simulink model "WK_Maobi_writingDTP25"  (Simulink 7.7)
settings: Solver=ode4  StartTime=0.0  StopTime=inf  FixedStep=sample_time  RelTol=1e-3
InitFcn:
  | sample_time=0.005;%0.004;%0.0025;%0.02;
  | DeltaT = 0.02;
  | g = 9.81;
  | H0 = g%0.3165;
  | Kl = 1;
  | 
  | Omega_r = 1.6;%for Horizontal reference
  | Zeta_r = 0.7; %for Horizontal reference
  | Omega = 1.8;%for Horizontal Control
  | Zeta = 0.5;    %for Horizontal Control
  | 
  | Omega_h_r = 2.5; %for vertical reference
  | Zeta_h_r = 0.8;  %for vertical reference
  | Omega_h = 2.7;    %for vertical control
  | Zeta_h = 0.8;         %for vertical control
  | PI=pi;
  | 
  | Mass = 1.15;
  | Acc_Max = 4;
  | Acc_Max_h = 4;
  | 
  | Max_RP = 60;
  | 
  | % for NN
  | n = 5;
  | r = 3;
  | n2 = 5;
  | NN_ST = 0.02;
  | 
  | GAMA_V = 6;
  | gama_V_e = 0.01;
  | 
  | GAMA_W = GAMA_V;
  | gama_W_e =0.01;
  | 
  | % deadzone
  | NN_Deadzone_Z = 0;
  | 
  | % inputs nomalizaton parameters
  | NN_Z_y_min = -3;
  | NN_Z_y_max = 0.5;
  | 
  | NN_Z_v_max = 8;
  | NN_Z_v_min = -NN_Z_v_max;
  | 
  | % alpha = 0.034;
  | alpha = 1;
  | % c_f = 0.0015;
  | c_f = 0.001;
  | c_y_tilt = 1*0.5;
  | 
  | %for WK paras
  | Heightcontrol = 0.08;
  | Scale_Factor=1;
  | yoffset=0;
  | 
  | load MaoBi_Oct04_2_int.mat
  | MB_Interp.time = [];
undefined symbols (not defined in the file or in its folder): DiscIntNeverNeededParam
libraries: simulink x7, dspadpt3 x3, X330_Control x2
(part 2 of 2)

== system WK_Maobi_writingDTP25/Vicon_Data/Raw Quad Pose from Vicon/Process Vicon Raw Data1/Flip_pi1/Flip_0_to_2pi ==
  Angle : Inport
  Add : Sum
  Compare To Constant1 : simulink/Logic and Bit Operations/Compare To Constant  SystemSampleTime=-1  relop=<  const=0  LogicOutDataTypeMode=uint8  ZeroCross=off
  Constant : Constant  Value=2*pi
  Data Type Duplicate : DataTypeDuplicate
  Flip_2pi : Subsystem
      mask Type: Flip -2pi to 2pi
      mask Description: Flips the inputs into the range -2pi to +2pi
      mask Help: Flips the inputs into the range -2pi to +2pi
      mask Display: disp('Flip_2pi')
  Switch : Switch  Criteria=u2 ~= 0
  Angle_Flip : Outport
  wires:
  Flip_2pi/1(Angle_Flip) -> Compare To Constant1/1, Add/2, Switch/3
  Compare To Constant1/1 -> Switch/2
  Constant/1 -> Add/1
  Add/1 -> Switch/1
  Angle/1 -> Flip_2pi/1(Angle), Data Type Duplicate/2
  Switch/1 -> Angle_Flip/1, Data Type Duplicate/1

== system WK_Maobi_writingDTP25/Vicon_Data/Raw Quad Pose from Vicon/Process Vicon Raw Data6/Flip_pi1/Flip_0_to_2pi ==
  Angle : Inport
  Add : Sum
  Compare To Constant1 : simulink/Logic and Bit Operations/Compare To Constant  SystemSampleTime=-1  relop=<  const=0  LogicOutDataTypeMode=uint8  ZeroCross=off
  Constant : Constant  Value=2*pi
  Data Type Duplicate : DataTypeDuplicate
  Flip_2pi : Subsystem
      mask Type: Flip -2pi to 2pi
      mask Description: Flips the inputs into the range -2pi to +2pi
      mask Help: Flips the inputs into the range -2pi to +2pi
      mask Display: disp('Flip_2pi')
  Switch : Switch  Criteria=u2 ~= 0
  Angle_Flip : Outport
  wires:
  Flip_2pi/1(Angle_Flip) -> Compare To Constant1/1, Add/2, Switch/3
  Compare To Constant1/1 -> Switch/2
  Constant/1 -> Add/1
  Add/1 -> Switch/1
  Angle/1 -> Flip_2pi/1(Angle), Data Type Duplicate/2
  Switch/1 -> Angle_Flip/1, Data Type Duplicate/1

== system WK_Maobi_writingDTP25/Vicon_Data/Raw Quad Pose from Vicon/Process Vicon Raw Data7/Flip_pi1/Flip_0_to_2pi ==
  Angle : Inport
  Add : Sum
  Compare To Constant1 : simulink/Logic and Bit Operations/Compare To Constant  SystemSampleTime=-1  relop=<  const=0  LogicOutDataTypeMode=uint8  ZeroCross=off
  Constant : Constant  Value=2*pi
  Data Type Duplicate : DataTypeDuplicate
  Flip_2pi : Subsystem
      mask Type: Flip -2pi to 2pi
      mask Description: Flips the inputs into the range -2pi to +2pi
      mask Help: Flips the inputs into the range -2pi to +2pi
      mask Display: disp('Flip_2pi')
  Switch : Switch  Criteria=u2 ~= 0
  Angle_Flip : Outport
  wires:
  Switch/1 -> Data Type Duplicate/1, Angle_Flip/1
  Angle/1 -> Data Type Duplicate/2, Flip_2pi/1(Angle)
  Add/1 -> Switch/1
  Constant/1 -> Add/1
  Compare To Constant1/1 -> Switch/2
  Flip_2pi/1(Angle_Flip) -> Switch/3, Add/2, Compare To Constant1/1

== system WK_Maobi_writingDTP25/Vicon_Data/Raw Quad Pose from Vicon/Process Vicon Raw Data1/Flip_pi1/Flip_0_to_2pi/Flip_2pi ==
  Angle : Inport
  Bias : Bias  Bias=-2*pi
  Constant : Constant  Value=2*pi
  Data Type Duplicate : DataTypeDuplicate
  Modulo : Math  Operator=mod  SaturateOnIntegerOverflow=on
  Sign1 : Signum
  Switch : Switch
  Angle_Flip : Outport
  wires:
  Angle/1 -> Modulo/1, Sign1/1, Data Type Duplicate/1
  Constant/1 -> Modulo/2
  Modulo/1 -> Bias/1, Switch/1
  Sign1/1 -> Switch/2
  Bias/1 -> Switch/3
  Switch/1 -> Angle_Flip/1, Data Type Duplicate/2

== system WK_Maobi_writingDTP25/Vicon_Data/Raw Quad Pose from Vicon/Process Vicon Raw Data6/Flip_pi1/Flip_0_to_2pi/Flip_2pi ==
  Angle : Inport
  Bias : Bias  Bias=-2*pi
  Constant : Constant  Value=2*pi
  Data Type Duplicate : DataTypeDuplicate
  Modulo : Math  Operator=mod  SaturateOnIntegerOverflow=on
  Sign1 : Signum
  Switch : Switch
  Angle_Flip : Outport
  wires:
  Angle/1 -> Modulo/1, Sign1/1, Data Type Duplicate/1
  Constant/1 -> Modulo/2
  Modulo/1 -> Bias/1, Switch/1
  Sign1/1 -> Switch/2
  Bias/1 -> Switch/3
  Switch/1 -> Angle_Flip/1, Data Type Duplicate/2

== system WK_Maobi_writingDTP25/Vicon_Data/Raw Quad Pose from Vicon/Process Vicon Raw Data7/Flip_pi1/Flip_0_to_2pi/Flip_2pi ==
  Angle : Inport
  Bias : Bias  Bias=-2*pi
  Constant : Constant  Value=2*pi
  Data Type Duplicate : DataTypeDuplicate
  Modulo : Math  Operator=mod  SaturateOnIntegerOverflow=on
  Sign1 : Signum
  Switch : Switch
  Angle_Flip : Outport
  wires:
  Switch/1 -> Data Type Duplicate/2, Angle_Flip/1
  Bias/1 -> Switch/3
  Sign1/1 -> Switch/2
  Modulo/1 -> Switch/1, Bias/1
  Constant/1 -> Modulo/2
  Angle/1 -> Data Type Duplicate/1, Sign1/1, Modulo/1

== matlab function Planning/Yaw Controller/MATLAB Function ==
  data: u input double; y output double
function y = fcn(u)
%#codegen
y = u;
if y > pi    
    y = y - 2*pi;
elseif y < -pi
        y = y + 2*pi;
end

== stateflow chart Planning/Trajectory Logic/UAV SF ==
  state Landing
    state Descending
      en:PosDesired = Pos;
      du:PosDesired[2] = (PerchPos[2]- PosDesired[2])*1*DeltaT + PosDesired[2] ;
    state CutThrottle
      du:HoverThrottle = (PerchPos[2] - HoverThrottle)*3*DeltaT + HoverThrottle ;
    (default) -> Descending
    Descending -> CutThrottle : [Pos[2] >(PerchPos[2] -0.1)]
  state Airborne
    state TakeOff
      du:HoverThrottle = (H0 - HoverThrottle)*3*DeltaT + HoverThrottle ;
    state Descent1
      descentrate=descentrate+0.02;
    state Descent
      en:PosDesired[2] = PerchPos[2]-0.50+descentrate;
    state Prelanding
      en:PosDesired[0] = PerchPos[0]; PosDesired[1] = PerchPos[1];PosDesired[2] = PerchPos[2]-0.8 ;
      descentrate=0;
    state SafyHover
      en:PosDesired = Pos; PosDesired[2]=-1.0;
    state D_Letter
      state drawing_straight_line
        en:
        PosDesired[0]=draw[0]-0.23, PosDesired[1]=draw[1]-0.1,PosDesired[2]= draw[2]-1.0;
        degree=-1.5707;
      state drawing_circle_line1
        en:
        PosDesired[0]=draw[0]-0.23, PosDesired[1]=draw[1]-0.1,PosDesired[2]= draw[2]-1.0;
      state MBdown
        en:
        PosDesired[0]=draw[0]-0.23, PosDesired[1]=draw[1]-0.1, PosDesired[2]=draw[2]-0.455
      state End_Point
        en:
        PosDesired[0]=draw[0]-0.23, PosDesired[1]=draw[1]+0.1,PosDesired[2]= draw[2]-0.455;
      state MBup
        en: PosDesired[2]= draw[2]-1.0;
      state End_Point1
        en:
        PosDesired[0]=draw[0]-0.23, PosDesired[1]=draw[1]+0.1,PosDesired[2]= draw[2]-0.455;
      state drawing_circle_line2
        en:
        degree= degree+0.08726;
        PosDesired[2]=draw[2]-0.455;
      state MBdown1
        en:
        PosDesired[0]=draw[0]-0.023+0.1*cos(degree);
        PosDesired[1]=draw[1]+0.1*sin(degree);
        PosDesired[2]=draw[2]-0.455
      state MBup1
        en:
        PosDesired[2]= draw[2]-1.0;
      (default) -> drawing_straight_line
      drawing_straight_line -> MBdown : [(abs(PosDesired[0]-draw[0]+0.23)+abs(PosDesired[1]-draw[1]+0.1)+abs(PosDesired[2]-draw[2]+1.0)) <0.02]
      MBup -> drawing_circle_line1 : [PosDesired[2]-draw[2]+1.0<0.01]
      MBdown1 -> drawing_circle_line2 [order 1] : [degree<3.1415]
      MBdown -> End_Point : [(abs(PosDesired[0]-draw[0]+0.23)+abs(PosDesired[1]-draw[1]+0.1)+abs(PosDesired[2]-draw[2]+0.455)) <0.02]
      End_Point -> MBup : [(abs(PosDesired[0]-draw[0]+0.23)+abs(PosDesired[1]-draw[1]+0.1)+abs(PosDesired[2]-draw[2]+0.455)) <0.02]
      End_Point1 -> MBup1 : [(abs(PosDesired[0]-draw[0]+0.23)+abs(PosDesired[1]-draw[1]-0.1)<0.02]
      MBdown1 -> End_Point1 [order 2] : [degree>3.1415]
      drawing_circle_line2 -> MBdown1 : after (1,sec)
      drawing_circle_line1 -> MBdown1 : [(abs(PosDesired[0]-draw[0]+0.23)+abs(PosDesired[1]-draw[1]+0.1)+abs(PosDesired[2]-draw[2]+1)) <0.02]
    state T_Letter
      state drawing_straight_line1
        en:
        PosDesired[0]=draw[0]-0.16, PosDesired[1]=draw[1]-0.1,PosDesired[2]= draw[2]-1.0;
      state MBdown2
        en:
        PosDesired[0]=draw[0]-0.16, PosDesired[1]=draw[1]-0.1, PosDesired[2]=draw[2]-0.455
      state End_Point2
        en:
        PosDesired[0]=draw[0]-0.06, PosDesired[1]=draw[1]-0.1,PosDesired[2]= draw[2]-0.455;
      state MBup2
        en: PosDesired[2]= draw[2]-1.0;
      state drawing_straight_line2
        en:
        PosDesired[0]=draw[0]-0.11, PosDesired[1]=draw[1]-0.1,PosDesired[2]= draw[2]-1.0;
      state MBdown3
        en:
        PosDesired[0]=draw[0]-0.11, PosDesired[1]=draw[1]-0.1, PosDesired[2]=draw[2]-0.455
      state Mid_Point
        en:
        PosDesired[0]=draw[0]-0.11, PosDesired[1]=draw[1],PosDesired[2]= draw[2]-0.455;
      state End_Point4
        en:
        PosDesired[0]=draw[0]-0.11, PosDesired[1]=draw[1]+0.1,PosDesired[2]= draw[2]-0.455;
      state MBup2
        en:
        PosDesired[2]= draw[2]-1.0;
      (default) -> Airborne.T_Letter.drawing_straight_line1
      Airborne.T_Letter.drawing_straight_line1 -> Airborne.T_Letter.MBdown2 : [(abs(PosDesired[0]-draw[0]+0.16)+abs(PosDesired[1]-draw[1]+0.1)+abs(PosDesired[2]-draw[2]+1.0)) <0.02]
      Airborne.T_Letter.MBdown2 -> Airborne.T_Letter.End_Point2 : [(abs(PosDesired[0]-draw[0]+0.16)+abs(PosDesired[1]-draw[1]+0.1)+abs(PosDesired[2]-draw[2]+0.455)) <0.02]
      Airborne.T_Letter.End_Point2 -> Airborne.T_Letter.MBup2 : [(abs(PosDesired[0]-draw[0]+0.06)+abs(PosDesired[1]-draw[1]+0.1)+abs(PosDesired[2]-draw[2]+0.455)) <0.02]
      Airborne.T_Letter.MBup2 -> Airborne.T_Letter.drawing_straight_line2 : [PosDesired[2]-draw[2]+1.0<0.01]
      Airborne.T_Letter.drawing_straight_line2 -> Airborne.T_Letter.MBdown3 : [(abs(PosDesired[0]-draw[0]+0.11)+abs(PosDesired[1]-draw[1]+0.1)+abs(PosDesired[2]-draw[2]+1.0)) <0.02]
      Airborne.T_Letter.MBdown3 -> Mid_Point : after(1,sec)
      Mid_Point -> Airborne.T_Letter.End_Point4 : [(abs(PosDesired[0]-draw[0]+0.11)+abs(PosDesired[1]-draw[1])+abs(PosDesired[2]-draw[2]+1.0)) <0.02]
      Airborne.T_Letter.End_Point4 -> Airborne.T_Letter.MBup2 : [(abs(PosDesired[0]-draw[0]+0.11)+abs(PosDesired[1]-draw[1]-0.1)<0.02]
    state P_Letter
      state drawing_straight_line1
        en:
        PosDesired[0]=draw[0]-0.04, PosDesired[1]=draw[1]-0.1,PosDesired[2]= draw[2]-1.0;
        degree=-1.5707;
      state MBdown2
        en:
        PosDesired[0]=draw[0]-0.04, PosDesired[1]=draw[1]-0.1, PosDesired[2]=draw[2]-0.455
      state End_Point2
        en:
        PosDesired[0]=draw[0]-0.04, PosDesired[1]=draw[1]+0.1,PosDesired[2]= draw[2]-0.455;
      state MBup3
        en: PosDesired[2]= draw[2]-1.0;
      state drawing_circle_line3
        en:
        PosDesired[0]=draw[0]-0.04, PosDesired[1]=draw[1]-0.1,PosDesired[2]= draw[2]-1.0;
      state MBdown2
        en:
        PosDesired[0]=draw[0]-0.04+0.05*cos(degree);
        PosDesired[1]=draw[1]-0.05+0.05*sin(degree);
        PosDesired[2]=draw[2]-0.455
      state drawing_circle_line3
        en:
        degree= degree+0.08726;
        PosDesired[2]=draw[2]-0.455;
      state End_Point2
        en:
        PosDesired[0]=draw[0]-0.04, PosDesired[1]=draw[1],PosDesired[2]= draw[2]-0.455;
      state MBup2
        en:
        PosDesired[2]= draw[2]-1.0;
      (default) -> Airborne.P_Letter.drawing_straight_line1
      Airborne.P_Letter.drawing_straight_line1 -> Airborne.P_Letter.MBdown2 : [(abs(PosDesired[0]-draw[0]+0.04)+abs(PosDesired[1]-draw[1]+0.1)+abs(PosDesired[2]-draw[2]+1.0)) <0.02]
      Airborne.P_Letter.MBdown2 -> Airborne.P_Letter.End_Point2 : [(abs(PosDesired[0]-draw[0]+0.04)+abs(PosDesired[1]-draw[1]+0.1)+abs(PosDesired[2]-draw[2]+0.455)) <0.02]
      Airborne.P_Letter.End_Point2 -> Airborne.P_Letter.MBup3 : [(abs(PosDesired[0]-draw[0]+0.04)+abs(PosDesired[1]-draw[1]-0.1)+abs(PosDesired[2]-draw[2]+0.455)) <0.02]
      Airborne.P_Letter.MBup3 -> Airborne.P_Letter.drawing_circle_line3 : [PosDesired[2]-draw[2]+1.0<0.01]
      Airborne.P_Letter.MBdown2 -> Airborne.P_Letter.drawing_circle_line3 [order 1] : [degree<3.1415]
      Airborne.P_Letter.drawing_circle_line3 -> Airborne.P_Letter.MBdown2 : after (1,sec)
      Airborne.P_Letter.MBdown2 -> Airborne.P_Letter.End_Point2 [order 2] : [degree>3.1415]
      Airborne.P_Letter.drawing_circle_line3 -> Airborne.P_Letter.MBdown2 : [(abs(PosDesired[0]-draw[0]+0.04)+abs(PosDesired[1]-draw[1]+0.1)+abs(PosDesired[2]-draw[2]+1.0)) <0.02]
      Airborne.P_Letter.End_Point2 -> Airborne.P_Letter.MBup2 : [(abs(PosDesired[0]-draw[0]+0.04))+abs(PosDesired[1]-draw[1])<0.02]
    state 2_Letter1
      state MBup3
        en: PosDesired[2]= draw[2]-1.0;
      state drawing_straight_line1
        en:
        PosDesired[0]=draw[0]+0.075, PosDesired[1]=draw[1]-0.05,PosDesired[2]= draw[2]-1.0;
        degree=3.1415;
      state MBdown3
        en:
        PosDesired[0]=draw[0]+0.075+0.05*cos(degree);
        PosDesired[1]=draw[1]-0.05+0.05*sin(degree);
        PosDesired[2]=draw[2]-0.455
      state drawing_circle_line4
        en:
        degree= degree+0.08726;
        PosDesired[2]=draw[2]-0.455;
      state End_Point3
        en:
        PosDesired[0]=draw[0]+0.125, PosDesired[1]=draw[1]-0.05,PosDesired[2]= draw[2]-0.455;
      state drawing_diagonal_line
        en:
        PosDesired[0]=draw[0]+0.125, PosDesired[1]=draw[1]-0.05,PosDesired[2]= draw[2]-1.0;
      state MBdown3
        en:
        PosDesired[0]=draw[0]+0.125, PosDesired[1]=draw[1]-0.05, PosDesired[2]=draw[2]-0.455
      state drawing_diagonal_line_mid
        en:
        PosDesired[0]=draw[0]+0.075, PosDesired[1]=draw[1]+0.025,PosDesired[2]= draw[2]-0.455;
      state drawing_diagonal_line_end
        en:
        PosDesired[0]=draw[0]+0.025, PosDesired[1]=draw[1]+0.1,PosDesired[2]= draw[2]-0.455;
      state drawing_straight_line2
        en:
        PosDesired[0]=draw[0]+0.025, PosDesired[1]=draw[1]+0.1,PosDesired[2]= draw[2]-1.0;
      state MBup4
        en: PosDesired[2]= draw[2]-1.0;
      state MBdown4
        en:
        PosDesired[0]=draw[0]+0.025, PosDesired[1]=draw[1]+0.1, PosDesired[2]=draw[2]-0.455
      state End_Point4
        en:
        PosDesired[0]=draw[0]+0.125, PosDesired[1]=draw[1]+0.1,PosDesired[2]= draw[2]-0.455;
      state MBup5
        en: PosDesired[2]= draw[2]-1.0;
      (default) -> Airborne.2_Letter1.drawing_straight_line1
      Airborne.2_Letter1.drawing_straight_line1 -> Airborne.2_Letter1.MBdown3 : [(abs(PosDesired[0]-draw[0]-0.075)+abs(PosDesired[1]-draw[1]+0.05)+abs(PosDesired[2]-draw[2]+1.0)) <0.02]
      drawing_circle_line4 -> Airborne.2_Letter1.MBdown3 : after (1,sec)
      Airborne.2_Letter1.MBdown3 -> drawing_circle_line4 [order 1] : [degree<6.283]
      End_Point3 -> Airborne.2_Letter1.MBup3 : [(abs(PosDesired[0]-draw[0]-0.125)+abs(PosDesired[1]-draw[1]+0.05)+abs(PosDesired[2]-draw[2]+0.455)) <0.02]
      Airborne.2_Letter1.MBdown3 -> End_Point3 [order 2] : [degee >6.283]
      Airborne.2_Letter1.MBup3 -> drawing_diagonal_line : [PosDesired[2]-draw[2]+1.0<0.01]
      drawing_diagonal_line -> Airborne.2_Letter1.MBdown3 : [(abs(PosDesired[0]-draw[0]-0.125)+abs(PosDesired[1]-draw[1]+0.05)+abs(PosDesired[2]-draw[2]+0.455)) <0.02]
      Airborne.2_Letter1.MBdown3 -> drawing_diagonal_line_mid : after(1,sec)
      drawing_diagonal_line_mid -> drawing_diagonal_line_end : after(1,sec)
      drawing_diagonal_line_end -> MBup4 : [(abs(PosDesired[0]-draw[0]-0.125)+abs(PosDesired[1]-draw[1]-0.1)+abs(PosDesired[2]-draw[2]+0.455)) <0.02]
      MBup4 -> Airborne.2_Letter1.drawing_straight_line2 : [abs(PosDesired[2]-draw[2]+1.0)<0.01]
      Airborne.2_Letter1.drawing_straight_line2 -> MBdown4 : [(abs(PosDesired[0]-draw[0]-0.025)+abs(PosDesired[1]-draw[1]-0.1)+abs(PosDesired[2]-draw[2]+1)) <0.02]
      MBdown4 -> Airborne.2_Letter1.End_Point4 : [(abs(PosDesired[0]-draw[0]-0.025)+abs(PosDesired[1]-draw[1]-0.1)+abs(PosDesired[2]-draw[2]+0.455)) <0.02]
      Airborne.2_Letter1.End_Point4 -> MBup5 : [(abs(PosDesired[0]-draw[0]-0.125)+abs(PosDesired[1]-draw[1]-0.1)+abs(PosDesired[2]-draw[2]+0.455)) <0.02]
    state 5_Letter
      state drawing_straight_line1
        en:
        PosDesired[0]=draw[0]+0.235, PosDesired[1]=draw[1]-0.1,PosDesired[2]= draw[2]-1.0;
      state MBdown5
        en:
        PosDesired[0]=draw[0]+0.235, PosDesired[1]=draw[1]-0.1, PosDesired[2]=draw[2]-0.455
      state drawing_straight_line_end1
        en:
        PosDesired[0]=draw[0]+0.145, PosDesired[1]=draw[1]-0.1,PosDesired[2]= draw[2]-0.455;
      state MBup6
        en: PosDesired[2]= draw[2]-1.0;
      state drawing_straight_line3
        en:
        PosDesired[0]=draw[0]+0.145, PosDesired[1]=draw[1]-0.1,PosDesired[2]= draw[2]-1.0;
      state MBdown6
        en:
        PosDesired[0]=draw[0]+0.145, PosDesired[1]=draw[1]-0.1, PosDesired[2]=draw[2]-0.455
      state drawing_straight_line_end2
        en:
        PosDesired[0]=draw[0]+0.145, PosDesired[1]=draw[1],PosDesired[2]= draw[2]-0.455;
      state MBup7
        en: PosDesired[2]= draw[2]-1.0;
      state drawing_straight_line5
        en:
        PosDesired[0]=draw[0]+0.145, PosDesired[1]=draw[1],PosDesired[2]= draw[2]-1.0;
      state MBdown7
        en:
        PosDesired[0]=draw[0]+0.145, PosDesired[1]=draw[1], PosDesired[2]=draw[2]-0.455
      state drawing_straight_line_end3
        en:
        PosDesired[0]=draw[0]+0.195, PosDesired[1]=draw[1],PosDesired[2]= draw[2]-0.455;
      state MBup8
        en: PosDesired[2]= draw[2]-1.0;
        degree=0;
      state MBdown5
        en:
        PosDesired[0]=draw[0]+0.195+0.05*cos(degree);
        PosDesired[1]=draw[1]+0.05+0.05*sin(degree);
        PosDesired[2]=draw[2]-0.455
      state drawing_circle_line5
        en:
        degree= degree+0.08726;
        PosDesired[2]=draw[2]-0.455;
      state End_Point5
        en:
        PosDesired[0]=draw[0]+0.195, PosDesired[1]=draw[1]-0.1,PosDesired[2]= draw[2]-0.455;
      state drawing_straight_line_end4
        en:
        PosDesired[0]=draw[0]+0.145, PosDesired[1]=draw[1]-0.1,PosDesired[2]= draw[2]-0.455;
      state MBup9
        en: PosDesired[2]= draw[2]-1.0;
      (default) -> Airborne.5_Letter.drawing_straight_line1
      Airborne.5_Letter.drawing_straight_line1 -> Airborne.5_Letter.MBdown5 : [(abs(PosDesired[0]-draw[0]-0.235)+abs(PosDesired[1]-draw[1]+0.1)+abs(PosDesired[2]-draw[2]+1.0)) <0.02]
      Airborne.5_Letter.MBdown5 -> drawing_straight_line_end1 : [(abs(PosDesired[0]-draw[0]-0.235)+abs(PosDesired[1]-draw[1]+0.1)+abs(PosDesired[2]-draw[2]+0.455)) <0.02]
      drawing_straight_line_end1 -> MBup6 : [(abs(PosDesired[0]-draw[0]-0.145)+abs(PosDesired[1]-draw[1]+0.1)+abs(PosDesired[2]-draw[2]+0.455)) <0.02]
      MBup6 -> drawing_straight_line3 : [abs(PosDesired[2]-draw[2]+1) <0.02]
      drawing_straight_line3 -> MBdown6 : [(abs(PosDesired[0]-draw[0]-0.145)+abs(PosDesired[1]-draw[1]+0.1)+abs(PosDesired[2]-draw[2]+1.0)) <0.02]
      MBdown6 -> drawing_straight_line_end2 : [abs(PosDesired[2]-draw[2]+0.455) <0.02]
      drawing_straight_line_end2 -> MBup7 : [(abs(PosDesired[0]-draw[0]-0.145)+abs(PosDesired[1]-draw[1])+abs(PosDesired[2]-draw[2]+0.455)) <0.02]
      MBup7 -> drawing_straight_line5 : [abs(PosDesired[2]-draw[2]+1) <0.02]
      drawing_straight_line5 -> MBdown7 : [(abs(PosDesired[0]-draw[0]-0.145)+abs(PosDesired[1]-draw[1])+abs(PosDesired[2]-draw[2]+1.0)) <0.02]
      MBdown7 -> drawing_straight_line_end3 : [abs(PosDesired[2]-draw[2]+0.455) <0.02]
      drawing_straight_line_end3 -> MBup8 : [(abs(PosDesired[0]-draw[0]-0.195)+abs(PosDesired[1]-draw[1])+abs(PosDesired[2]-draw[2]+0.455)) <0.02]
      MBup8 -> Airborne.5_Letter.MBdown5 : [abs(PosDesired[2]-draw[2]+0.455) <0.02]
      Airborne.5_Letter.MBdown5 -> drawing_circle_line5 [order 1] : [degree<3.1415]
      drawing_circle_line5 -> Airborne.5_Letter.MBdown5 : after(1,seec)
      Airborne.5_Letter.MBdown5 -> End_Point5 [order 2] : [degree>3.1415]
      End_Point5 -> drawing_straight_line_end4 : [(abs(PosDesired[0]-draw[0]-0.195)+abs(PosDesired[1]-draw[1]+0.1)+abs(PosDesired[2]-draw[2]+0.455)) <0.02]
      drawing_straight_line_end4 -> MBup9 : [(abs(PosDesired[0]-draw[0]-0.145)+abs(PosDesired[1]-draw[1]+0.1)+abs(PosDesired[2]-draw[2]+0.455)) <0.02]
    state SafyHover1
      en:PosDesired = Pos; PosDesired[2]=-1.0;
    Descent -> Prelanding [order 1] : after (5,sec)
    (default) -> TakeOff : {PosDesired = Pos;  PosDesired[2] =-1.2;}
    SafyHover -> Prelanding : after (3, sec)
    Descent1 -> Descent : after (0.5,sec)
    Prelanding -> Descent : [PerchError < 0.01]
    Descent -> Descent1 [order 2] : [PerchError < 0.02]
    TakeOff -> SafyHover [order 2] : [RC[5] > 0.5]
    D_Letter -> SafyHover [order 3] : [RC[5] > 0.5]
    TakeOff -> D_Letter [order 1] : after (5,sec)
    D_Letter -> T_Letter [order 1] : [(abs(PosDesired[0]-draw[0]+0.23)+abs(PosDesired[1]-draw[1]-0.1)+abs(PosDesired[2]-draw[2]+1.0)) <0.02]
    T_Letter -> P_Letter [order 1] : [(abs(PosDesired[0]-draw[0]+0.11)+abs(PosDesired[1]-draw[1]-0.1)+abs(PosDesired[2]-draw[2]+1.0)) <0.02]
    P_Letter -> 2_Letter1 [order 1] : [(abs(PosDesired[0]-draw[0]+0.11)+abs(PosDesired[1]-draw[1]-0.1)+abs(PosDesired[2]-draw[2]+1.0)) <0.02]
    2_Letter1 -> 5_Letter [order 1] : [(abs(PosDesired[0]-draw[0]-0.125)+abs(PosDesired[1]-draw[1]-0.1)+abs(PosDesired[2]-draw[2]+1.0)) <0.02]
    SafyHover1 -> Prelanding : after(3,sec)
    D_Letter -> SafyHover1 [order 2] : [RC[5] > 0.5]
    T_Letter -> SafyHover1 [order 2] : [RC[5] > 0.5]
    P_Letter -> SafyHover1 [order 2] : [RC[5] > 0.5]
    2_Letter1 -> SafyHover1 [order 2] : [RC[5] > 0.5]
  (default) -> Landing : {HoverThrottle = 0;}
  Airborne -> Landing : [RC[6] < -0.5]
  Landing -> Airborne : [RC[6] > 0.5]
  5_Letter -> SafyHover1 : [RC[5] > 0.5]
  data: PosDesired output double size=4; HoverThrottle output double size=1; Mode output uint8 size=1; RC input double size=8; Pos input double size=4; PerchPos input double size=4; DeltaT parameter double size=1; H0 parameter double size=1; Kl parameter double size=1; VelCmd local double size=2 =0; PWM output double; PerchError input double; PI parameter double size=1; draw input double size=3; descentrate local double; degree local double
